simulink model "VehCo_VehDem"  (R2018a)
settings: configuration reference "cs_ert" (kept outside this file)
settings Model: DataDictionary=VehCo_VehDem.sldd  Creator=zhoutinglin  LastModifiedBy=zhoutinglin

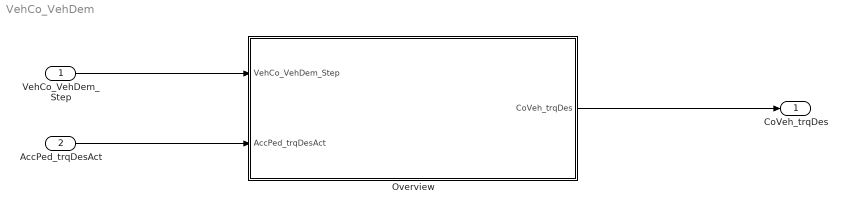
== system VehCo_VehDem ==
  VehCo_VehDem_Step : Inport  OutputFunctionCall=on
  AccPed_trqDesAct : Inport  Description=driver torque raw of propulsion  Port=2  OutMin=-3000  OutMax=3000  OutDataTypeStr=Torq  Unit=Nm  PortDimensions=[1 1]
  Overview : Subsystem
  CoVeh_trqDes : Outport  Description=Setpoint torque order to the drive train (gearbox output torque)  OutMin=-3000  OutMax=3000  OutDataTypeStr=Torq  Unit=Nm  PortDimensions=[1 1]
  wires:
  VehCo_VehDem_Step/1 -> Overview/1(VehCo_VehDem_Step)
  AccPed_trqDesAct/1 -> Overview/2(AccPed_trqDesAct)
  Overview/1(CoVeh_trqDes) -> CoVeh_trqDes/1

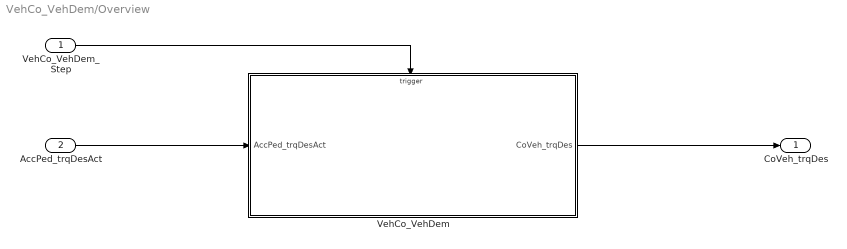
== system VehCo_VehDem/Overview ==
  VehCo_VehDem_Step : Inport
  AccPed_trqDesAct : Inport  Port=2
  VehCo_VehDem : Subsystem
  CoVeh_trqDes : Outport
  wires:
  AccPed_trqDesAct/1 -> VehCo_VehDem/1(AccPed_trqDesAct)
  VehCo_VehDem/1(CoVeh_trqDes) -> CoVeh_trqDes/1
  VehCo_VehDem_Step/1 -> VehCo_VehDem/Trigger

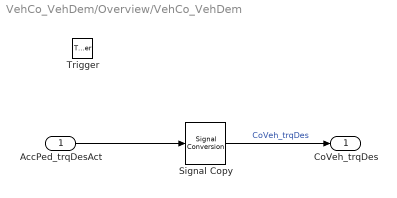
== system VehCo_VehDem/Overview/VehCo_VehDem ==
  AccPed_trqDesAct : Inport  Tag=Nm
  Trigger : TriggerPort  TriggerType=function-call  VariantControl=Variant  PortDimensions=1
  Signal Copy : SignalConversion  OverrideOpt=off
  CoVeh_trqDes : Outport  Tag=Nm
  wires:
  Signal Copy/1 -> CoVeh_trqDes/1  "CoVeh_trqDes"
  AccPed_trqDesAct/1 -> Signal Copy/1
